simulink model "quad_new_leg_raibert_strategy_v2"  (R2022b)
settings: Solver=ode15s  StartTime=0.0  StopTime=40  RelTol=1e-3
InitFcn:
  | init_quad_new_leg_raibert_strategy_v2
undefined symbols (not defined in the file): body, ctrl, Extr_Data_LinkEndHole, ground, l1, l2, m1, m2, planner, X, Y, Z
libraries: sm_lib x114, nesl_utility x74, slpidlib x24, simulink x5, Contact_Forces_Lib x4, Parts_Lib x4, sharedtransform x2
(part 1 of 7)
settings Model: Creator=biorobotics  LastModifiedBy=sheri
settings SolverCC: AlgebraicLoopSolver=TrustRegion
settings DataIOCC: ReturnWorkspaceOutputs=off
settings DebuggingCC: UnconnectedInputMsg=warning  UnconnectedOutputMsg=warning  UnconnectedLineMsg=warning  SFMachineParentedDataDiag=warning  ArithmeticOperatorsInVariantConditions=warning
settings ModelReferenceCC: EnableRefExpFcnMdlSchedulingChecks=on
settings SFSimCC: SimUseLocalCustomCode=off  CustomCodeUndefinedFunction=UseInterfaceOnly
settings RTWCC: RTWUseLocalCustomCode=off
settings DiagnosticsConfigSet: SimMechanicsRigidlyBoundBlock=none

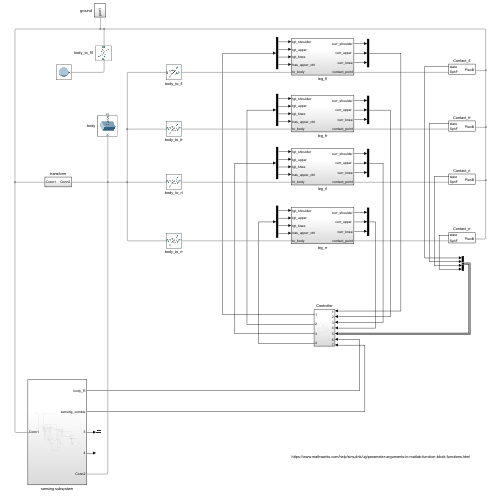
[thumbnail: Simulink's stored preview of the top-level diagram]
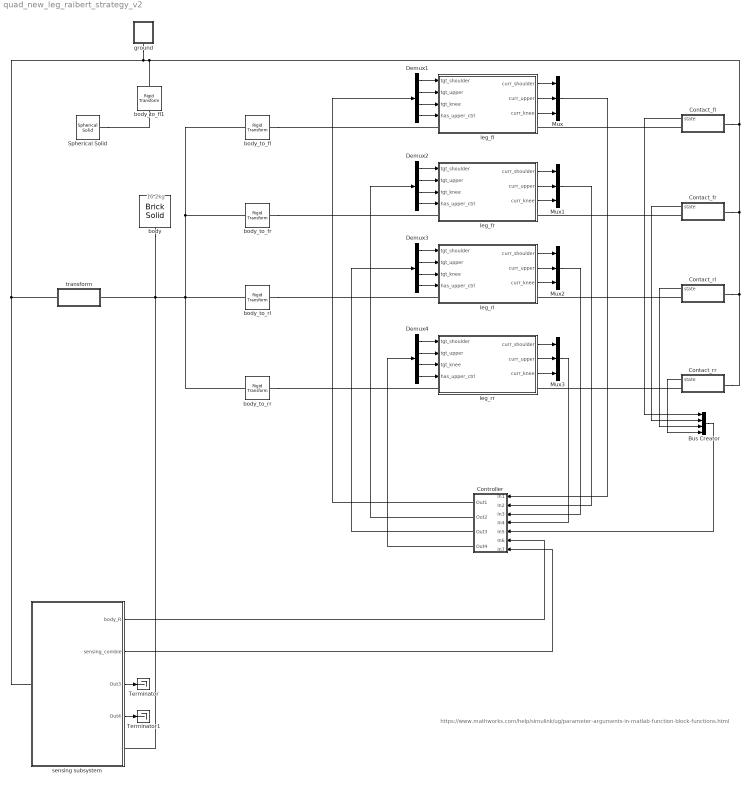
== system quad_new_leg_raibert_strategy_v2 ==
  note: https://www.mathworks.com/help/simulink/ug/parameter-arguments-in-matlab-function-block-functions.html
  note: 16.2kg
  Bus Creator : BusCreator  Inputs=4
  Contact_fl : Subsystem
  Contact_fr : Subsystem
  Contact_rl : Subsystem
  Contact_rr : Subsystem
  Controller : Subsystem
  Demux{1..4} (4 alike) : Demux
  Mux{,1..3} (4 alike) : Mux  Inputs=3
  Spherical Solid : sm_lib/Body Elements/Spherical Solid  GraphicAmbientColor=[0.15 0.15 0.15 1.0]  BasedOnType=Density  CenterOfMass=[0 0 0]  CenterOfMassUnits=m  GraphicDiffuseColor=[0.4 0.2 0.0]  Density=1000  DensityUnits=kg/m^3  DoExposeReferenceFrame=on  GraphicEmissiveColor=[0.0 0.0 0.0 1.0]  ExportEntireGeometry=off  SerializedExposedGeometries=<ExposedGeometries/>  SerializedFrames=<Frames/>  MarkerShape=Sphere  MarkerSize=10  GraphicType=FromGeometry  InertiaType=CalculateFromGeometry  Mass=1  MassUnits=kg  MomentsOfInertia=[1 1 1]  MomentsOfInertiaUnits=kg*m^2  GraphicOpacity=1.0  ProductsOfInertia=[0 0 0]  ProductsOfInertiaUnits=kg*m^2  GraphicShininess=75  GraphicSpecularColor=[0.5 0.5 0.5 1.0]  SphereRadius=0.1  SphereRadiusUnits=m  GraphicVisPropType=SimpleVisualProperties
  Terminator : Terminator
  Terminator1 : Terminator
  body : sm_lib/Body Elements/Brick Solid  GraphicAmbientColor=[0.15 0.15 0.15 1.0]  BasedOnType=Density  BrickDimensions=[body.x_length body.y_length body.z_length]  BrickDimensionUnits=m  CenterOfMass=[0 0 0]  CenterOfMassUnits=m  GraphicDiffuseColor=[164 184 200]/255  Density=600  DensityUnits=kg/(m^3)  DoExposeReferenceFrame=on  GraphicEmissiveColor=[0.0 0.0 0.0 1.0]  ExportEntireGeometry=off  SerializedFrames=<Frames><Frame><Id>Frame2</Id><Value><Name>force</Name><Origin><Source>CenterOfMassFrame</Source><FeatureName></FeatureName></Origin><PrimaryAxis><DefinedDirection>+Z</DefinedDirection><Source>ReferenceFrame</Source><SourceDirection>+Z</SourceDirection><FeatureName></FeatureName></PrimaryAxis><SecondaryAxis><DefinedDirection>+X</DefinedDirection><Source>ReferenceFrame</Source><SourceDirection>+X</SourceDirection><FeatureName></FeatureName></SecondaryAxis></Value></Frame></Frames>  MarkerShape=Sphere  MarkerSize=10  GraphicType=FromGeometry  InertiaType=CalculateFromGeometry  Mass=8.6  MassUnits=kg  MomentsOfInertia=[1 1 1]  MomentsOfInertiaUnits=kg*m^2  GraphicOpacity=1.0  ProductsOfInertia=[0 0 0]  ProductsOfInertiaUnits=kg*m^2  GraphicShininess=75  GraphicSpecularColor=[0.5 0.5 0.5 1.0]  GraphicVisPropType=SimpleVisualProperties
  body_to_fl : sm_lib/Frames and Transforms/Rigid Transform  TranslationMethod=Cartesian  TranslationStandardOffset=0  TranslationLengthUnit=m  TranslationStandardAxis=+Z  TranslationCartesianOffset=[body.shoulder_distance body.y_length/2+body.shoulder_size/2 0]  TranslationROffset=0  TranslationROffsetUnits=m  TranslationZOffset=0  TranslationZOffsetUnits=m  TranslationThetaOffset=0  TranslationThetaOffsetUnits=deg  RotationMethod=AlignedAxes  RotationAngleUnits=deg  RotationStandardAxis=+Z  RotationAngle=0.0  RotationArbitraryAxis=[0 0 1]  FollAlignAxisA=+Z  BaseAlignAxisA=+X  FollAlignAxisB=+X  BaseAlignAxisB=-Z  RotationSequenceAxes=FollowerAxes  RotationSequence=XYX  RotationSequenceAngles=[0 0 0]  RotationSequenceAnglesUnits=deg  RotationMatrix=[1 0 0; 0 1 0; 0 0 1]  Quaternion=[1 0 0 0]
  body_to_fl1 : sm_lib/Frames and Transforms/Rigid Transform  TranslationMethod=Cartesian  TranslationStandardOffset=0  TranslationLengthUnit=m  TranslationStandardAxis=+Z  TranslationCartesianOffset=[5 5 0]  TranslationROffset=0  TranslationROffsetUnits=m  TranslationZOffset=0  TranslationZOffsetUnits=m  TranslationThetaOffset=0  TranslationThetaOffsetUnits=deg  RotationMethod=None  RotationAngleUnits=deg  RotationStandardAxis=+Z  RotationAngle=0.0  RotationArbitraryAxis=[0 0 1]  FollAlignAxisA=+Z  BaseAlignAxisA=+X  FollAlignAxisB=+X  BaseAlignAxisB=-Z  RotationSequenceAxes=FollowerAxes  RotationSequence=XYX  RotationSequenceAngles=[0 0 0]  RotationSequenceAnglesUnits=deg  RotationMatrix=[1 0 0; 0 1 0; 0 0 1]  Quaternion=[1 0 0 0]
  body_to_fr : sm_lib/Frames and Transforms/Rigid Transform  TranslationMethod=Cartesian  TranslationStandardOffset=0  TranslationLengthUnit=m  TranslationStandardAxis=+Z  TranslationCartesianOffset=[body.shoulder_distance -body.y_length/2-body.shoulder_size/2 0]  TranslationROffset=0  TranslationROffsetUnits=m  TranslationZOffset=0  TranslationZOffsetUnits=m  TranslationThetaOffset=0  TranslationThetaOffsetUnits=deg  RotationMethod=AlignedAxes  RotationAngleUnits=deg  RotationStandardAxis=+Z  RotationAngle=0.0  RotationArbitraryAxis=[0 0 1]  FollAlignAxisA=+Z  BaseAlignAxisA=+X  FollAlignAxisB=+X  BaseAlignAxisB=-Z  RotationSequenceAxes=FollowerAxes  RotationSequence=XYX  RotationSequenceAngles=[0 0 0]  RotationSequenceAnglesUnits=deg  RotationMatrix=[1 0 0; 0 1 0; 0 0 1]  Quaternion=[1 0 0 0]
  body_to_rl : sm_lib/Frames and Transforms/Rigid Transform  TranslationMethod=Cartesian  TranslationStandardOffset=0  TranslationLengthUnit=m  TranslationStandardAxis=+Z  TranslationCartesianOffset=[-body.shoulder_distance body.y_length/2+body.shoulder_size/2 0]  TranslationROffset=0  TranslationROffsetUnits=m  TranslationZOffset=0  TranslationZOffsetUnits=m  TranslationThetaOffset=0  TranslationThetaOffsetUnits=deg  RotationMethod=AlignedAxes  RotationAngleUnits=deg  RotationStandardAxis=+Z  RotationAngle=0.0  RotationArbitraryAxis=[0 0 1]  FollAlignAxisA=+Z  BaseAlignAxisA=+X  FollAlignAxisB=+X  BaseAlignAxisB=-Z  RotationSequenceAxes=FollowerAxes  RotationSequence=XYX  RotationSequenceAngles=[0 0 0]  RotationSequenceAnglesUnits=deg  RotationMatrix=[1 0 0; 0 1 0; 0 0 1]  Quaternion=[1 0 0 0]
  body_to_rr : sm_lib/Frames and Transforms/Rigid Transform  TranslationMethod=Cartesian  TranslationStandardOffset=0  TranslationLengthUnit=m  TranslationStandardAxis=+Z  TranslationCartesianOffset=[-body.shoulder_distance -body.y_length/2-body.shoulder_size/2 0]  TranslationROffset=0  TranslationROffsetUnits=m  TranslationZOffset=0  TranslationZOffsetUnits=m  TranslationThetaOffset=0  TranslationThetaOffsetUnits=deg  RotationMethod=AlignedAxes  RotationAngleUnits=deg  RotationStandardAxis=+Z  RotationAngle=0.0  RotationArbitraryAxis=[0 0 1]  FollAlignAxisA=+Z  BaseAlignAxisA=+X  FollAlignAxisB=+X  BaseAlignAxisB=-Z  RotationSequenceAxes=FollowerAxes  RotationSequence=XYX  RotationSequenceAngles=[0 0 0]  RotationSequenceAnglesUnits=deg  RotationMatrix=[1 0 0; 0 1 0; 0 0 1]  Quaternion=[1 0 0 0]
  ground : Subsystem
  leg_fl : Subsystem
  leg_fr : Subsystem
  leg_rl : Subsystem
  leg_rr : Subsystem
  "sensing subsystem " : Subsystem
  transform : Subsystem
  wires:
  leg_fl/1(curr_shoulder) -> Mux/1
  leg_fl/2("curr_upper ") -> Mux/2
  leg_fl/3(curr_knee) -> Mux/3
  leg_fr/2("curr_upper ") -> Mux1/2
  leg_fr/1(curr_shoulder) -> Mux1/1
  leg_fr/3(curr_knee) -> Mux1/3
  leg_rl/1(curr_shoulder) -> Mux2/1
  leg_rl/2("curr_upper ") -> Mux2/2
  leg_rl/3(curr_knee) -> Mux2/3
  leg_rr/1(curr_shoulder) -> Mux3/1
  leg_rr/2("curr_upper ") -> Mux3/2
  leg_rr/3(curr_knee) -> Mux3/3
  Contact_fl/1(state) -> Bus Creator/1
  Contact_rr/1(state) -> Bus Creator/4
  Contact_rl/1(state) -> Bus Creator/3
  Contact_fr/1(state) -> Bus Creator/2
  Demux1/1 -> leg_fl/1(tgt_shoulder)
  Demux1/3 -> leg_fl/3(tgt_knee)
  Demux1/2 -> leg_fl/2(tgt_upper)
  Demux1/4 -> leg_fl/4(has_upper_ctrl)
  Demux2/1 -> leg_fr/1(tgt_shoulder)
  Demux2/3 -> leg_fr/3(tgt_knee)
  Demux2/4 -> leg_fr/4(has_upper_ctrl)
  Demux2/2 -> leg_fr/2(tgt_upper)
  Demux3/4 -> leg_rl/4(has_upper_ctrl)
  Demux3/3 -> leg_rl/3(tgt_knee)
  Demux3/1 -> leg_rl/1(tgt_shoulder)
  Demux3/2 -> leg_rl/2(tgt_upper)
  Demux4/1 -> leg_rr/1(tgt_shoulder)
  Demux4/2 -> leg_rr/2(tgt_upper)
  Demux4/3 -> leg_rr/3(tgt_knee)
  Demux4/4 -> leg_rr/4(has_upper_ctrl)
  Mux/1 -> Controller/1(In1)
  Mux1/1 -> Controller/2(In2)
  Mux2/1 -> Controller/3(In3)
  Mux3/1 -> Controller/4(In4)
  Bus Creator/1 -> Controller/5(In5)
  "sensing subsystem "/1(body_R) -> Controller/6(In6)
  "sensing subsystem "/2(sensing_combie) -> Controller/7(In7)
  Controller/1(Out1) -> Demux1/1
  Controller/2(Out2) -> Demux2/1
  Controller/3(Out3) -> Demux3/1
  Controller/4(Out4) -> Demux4/1
  "sensing subsystem "/3(Out3) -> Terminator/1
  "sensing subsystem "/4(Out4) -> Terminator1/1
  connections:
  body_to_fl/RConn1 -- leg_fl/LConn1
  body_to_rl/RConn1 -- leg_rl/LConn1
  Contact_fl/RConn1 -- leg_fl/RConn1
  Contact_fr/RConn1 -- leg_fr/RConn1
  Contact_rl/RConn1 -- leg_rl/RConn1
  Contact_rr/RConn1 -- leg_rr/RConn1
  body_to_rr/RConn1 -- leg_rr/LConn1
  body_to_fr/RConn1 -- leg_fr/LConn1
  Spherical Solid/RConn1 -- body_to_fl1/RConn1
  Contact_fr/LConn1 -- body_to_fl1/LConn1 -- transform/RConn1 -- "sensing subsystem "/LConn1 -- ground/RConn1 -- Contact_fl/LConn1 -- Contact_rr/LConn1 -- Contact_rl/LConn1
  body_to_rl/LConn1 -- body_to_rr/LConn1 -- body_to_fl/LConn1 -- body_to_fr/LConn1 -- transform/LConn1 -- body/RConn1 -- "sensing subsystem "/RConn1

== system quad_new_leg_raibert_strategy_v2/Contact_fl ==
  note: state 4 166.31ms
  note: 这是一个蛋疼的处理，因为地面现在厚度是0.4，为了和碰撞的block要求匹配，所以碰撞是相对于这个地面的中心来算的。而检测高度的时候就要把这个厚度减掉
      | 但是Transform sensor要检测的是球和地面的高度差
  Bus Selector : BusSelector  OutputSignals=Normal Force,Frame Sep,Friction Force
  Compare To Constant : simulink/Logic and Bit Operations/Compare To Constant  relop=<=  const=planner.touch_down_height  OutDataTypeStr=uint8
  PSConv4 : nesl_utility/PS-Simulink Converter  PhysicalDomain=network_engine_domain  SubClassName=ps_output  LeftPortType=input  RightPortType=output  PseudoPeriodic=off  Frequencies=[]  VectorFormat=1-D array  Unit=1  AffineConversion=off
  Sphere to Plane Force1 : Contact_Forces_Lib/3D/Sphere to Plane Force  sphere_rad=body.foot_radius  plane_lenx=12  plane_leny=12  plane_depth=0  force_law=Linear  k_contact=ground.stiff  b_contact=ground.damp  pen_full_damp_F=1e-4  pen_exponent=1  custom_param_1=1  custom_param_2=1  friction_law=Stick-Slip Continuous  mu_kinetic=0.7  mu_static=0.7  v_thr=0.001
  State Scope : Scope
  Terminator : Terminator
  Transform Sensor : sm_lib/Frames and Transforms/Transform Sensor  MeasurementFrame=World  SenseAngle=off  SenseAxis=off  SenseQ=off  SenseR=off  SenseRotationSequence=off  RotationSequence=XYX  SenseOmegaX=off  SenseOmegaY=off  SenseOmegaZ=off  SenseQDot=off  SenseRDot=off  SenseAlphaX=off  SenseAlphaY=off  SenseAlphaZ=off  SenseQDDot=off  SenseRDDot=off  SenseX=off  SenseY=off  SenseZ=on  SenseRad=off  SenseAzim=off  SenseDist=off  SenseInc=off  SenseXDot=off  SenseYDot=off  SenseZDot=off  SenseRadDot=off  SenseAzimDot=off  SenseDistDot=off  SenseIncDot=off  SenseXDDot=off  SenseYDDot=off  SenseZDDot=off  SenseRadDDot=off  SenseAzimDDot=off  SenseDistDDot=off  SenseIncDDot=off
  ZScope : Scope
  force : Scope  NumInputPorts=2
  PlanB : PMIOPort  Side=Left
  SphF : PMIOPort  Port=2  Side=Right
  state : Outport  VectorParamsAs1DForOutWhenUnconnected=off
  wires:
  Sphere to Plane Force1/1 -> Bus Selector/1
  Bus Selector/1 -> force/1  "<Normal Force>"
  PSConv4/1 -> Compare To Constant/1, ZScope/1
  Compare To Constant/1 -> state/1, State Scope/1
  Bus Selector/3 -> force/2  "<Friction Force>"
  Bus Selector/2 -> Terminator/1  "<Frame Sep>"
  connections:
  Sphere to Plane Force1/LConn1 -- Transform Sensor/RConn1 -- SphF/RConn1
  Sphere to Plane Force1/RConn1 -- Transform Sensor/LConn1 -- PlanB/RConn1
  PSConv4/LConn1 -- Transform Sensor/RConn2

== system quad_new_leg_raibert_strategy_v2/Contact_fr ==
  note: state 4 166.31ms
  note: 这是一个蛋疼的处理，因为地面现在厚度是0.4，为了和碰撞的block要求匹配，所以碰撞是相对于这个地面的中心来算的。而检测高度的时候就要把这个厚度减掉
      | 但是Transform sensor要检测的是球和地面的高度差
  Bus Selector : BusSelector  OutputSignals=Normal Force,Frame Sep,Friction Force
  Compare To Constant : simulink/Logic and Bit Operations/Compare To Constant  relop=<=  const=planner.touch_down_height  OutDataTypeStr=uint8
  PSConv4 : nesl_utility/PS-Simulink Converter  PhysicalDomain=network_engine_domain  SubClassName=ps_output  LeftPortType=input  RightPortType=output  PseudoPeriodic=off  Frequencies=[]  VectorFormat=1-D array  Unit=1  AffineConversion=off
  Sphere to Plane Force1 : Contact_Forces_Lib/3D/Sphere to Plane Force  sphere_rad=body.foot_radius  plane_lenx=12  plane_leny=12  plane_depth=0  force_law=Linear  k_contact=ground.stiff  b_contact=ground.damp  pen_full_damp_F=1e-4  pen_exponent=1  custom_param_1=1  custom_param_2=1  friction_law=Stick-Slip Continuous  mu_kinetic=0.7  mu_static=0.7  v_thr=0.001
  State Scope : Scope
  Terminator : Terminator
  Transform Sensor : sm_lib/Frames and Transforms/Transform Sensor  MeasurementFrame=World  SenseAngle=off  SenseAxis=off  SenseQ=off  SenseR=off  SenseRotationSequence=off  RotationSequence=XYX  SenseOmegaX=off  SenseOmegaY=off  SenseOmegaZ=off  SenseQDot=off  SenseRDot=off  SenseAlphaX=off  SenseAlphaY=off  SenseAlphaZ=off  SenseQDDot=off  SenseRDDot=off  SenseX=off  SenseY=off  SenseZ=on  SenseRad=off  SenseAzim=off  SenseDist=off  SenseInc=off  SenseXDot=off  SenseYDot=off  SenseZDot=off  SenseRadDot=off  SenseAzimDot=off  SenseDistDot=off  SenseIncDot=off  SenseXDDot=off  SenseYDDot=off  SenseZDDot=off  SenseRadDDot=off  SenseAzimDDot=off  SenseDistDDot=off  SenseIncDDot=off
  ZScope : Scope
  force : Scope  NumInputPorts=2
  PlanB : PMIOPort  Side=Left
  SphF : PMIOPort  Port=2  Side=Right
  state : Outport  VectorParamsAs1DForOutWhenUnconnected=off
  wires:
  Sphere to Plane Force1/1 -> Bus Selector/1
  Bus Selector/1 -> force/1  "<Normal Force>"
  PSConv4/1 -> Compare To Constant/1, ZScope/1
  Compare To Constant/1 -> state/1, State Scope/1
  Bus Selector/3 -> force/2  "<Friction Force>"
  Bus Selector/2 -> Terminator/1  "<Frame Sep>"
  connections:
  Sphere to Plane Force1/LConn1 -- Transform Sensor/RConn1 -- SphF/RConn1
  Sphere to Plane Force1/RConn1 -- Transform Sensor/LConn1 -- PlanB/RConn1
  PSConv4/LConn1 -- Transform Sensor/RConn2

== system quad_new_leg_raibert_strategy_v2/Contact_rl ==
  note: 这是一个蛋疼的处理，因为地面现在厚度是0.4，为了和碰撞的block要求匹配，所以碰撞是相对于这个地面的中心来算的。而检测高度的时候就要把这个厚度减掉
      | 但是Transform sensor要检测的是球和地面的高度差
  Bus Selector : BusSelector  OutputSignals=Normal Force,Frame Sep,Friction Force
  Compare To Constant : simulink/Logic and Bit Operations/Compare To Constant  relop=<=  const=planner.touch_down_height  OutDataTypeStr=uint8
  PSConv4 : nesl_utility/PS-Simulink Converter  PhysicalDomain=network_engine_domain  SubClassName=ps_output  LeftPortType=input  RightPortType=output  PseudoPeriodic=off  Frequencies=[]  VectorFormat=1-D array  Unit=1  AffineConversion=off
  Sphere to Plane Force1 : Contact_Forces_Lib/3D/Sphere to Plane Force  sphere_rad=body.foot_radius  plane_lenx=12  plane_leny=12  plane_depth=0  force_law=Linear  k_contact=ground.stiff  b_contact=ground.damp  pen_full_damp_F=1e-4  pen_exponent=1  custom_param_1=1  custom_param_2=1  friction_law=Stick-Slip Continuous  mu_kinetic=0.7  mu_static=0.7  v_thr=0.001
  State Scope : Scope
  Terminator : Terminator
  Transform Sensor : sm_lib/Frames and Transforms/Transform Sensor  MeasurementFrame=World  SenseAngle=off  SenseAxis=off  SenseQ=off  SenseR=off  SenseRotationSequence=off  RotationSequence=XYX  SenseOmegaX=off  SenseOmegaY=off  SenseOmegaZ=off  SenseQDot=off  SenseRDot=off  SenseAlphaX=off  SenseAlphaY=off  SenseAlphaZ=off  SenseQDDot=off  SenseRDDot=off  SenseX=off  SenseY=off  SenseZ=on  SenseRad=off  SenseAzim=off  SenseDist=off  SenseInc=off  SenseXDot=off  SenseYDot=off  SenseZDot=off  SenseRadDot=off  SenseAzimDot=off  SenseDistDot=off  SenseIncDot=off  SenseXDDot=off  SenseYDDot=off  SenseZDDot=off  SenseRadDDot=off  SenseAzimDDot=off  SenseDistDDot=off  SenseIncDDot=off
  ZScope : Scope
  force : Scope  NumInputPorts=2
  PlanB : PMIOPort  Side=Left
  SphF : PMIOPort  Port=2  Side=Right
  state : Outport  VectorParamsAs1DForOutWhenUnconnected=off
  wires:
  Sphere to Plane Force1/1 -> Bus Selector/1
  Bus Selector/1 -> force/1  "<Normal Force>"
  PSConv4/1 -> Compare To Constant/1, ZScope/1
  Compare To Constant/1 -> state/1, State Scope/1
  Bus Selector/3 -> force/2  "<Friction Force>"
  Bus Selector/2 -> Terminator/1  "<Frame Sep>"
  connections:
  Sphere to Plane Force1/LConn1 -- Transform Sensor/RConn1 -- SphF/RConn1
  Sphere to Plane Force1/RConn1 -- Transform Sensor/LConn1 -- PlanB/RConn1
  PSConv4/LConn1 -- Transform Sensor/RConn2

== system quad_new_leg_raibert_strategy_v2/Contact_rr ==
  note: state 4 166.31ms
  note: 这是一个蛋疼的处理，因为地面现在厚度是0.4，为了和碰撞的block要求匹配，所以碰撞是相对于这个地面的中心来算的。而检测高度的时候就要把这个厚度减掉
      | 但是Transform sensor要检测的是球和地面的高度差
  Bus Selector : BusSelector  OutputSignals=Normal Force,Frame Sep,Friction Force
  Compare To Constant : simulink/Logic and Bit Operations/Compare To Constant  relop=<=  const=planner.touch_down_height  OutDataTypeStr=uint8
  PSConv4 : nesl_utility/PS-Simulink Converter  PhysicalDomain=network_engine_domain  SubClassName=ps_output  LeftPortType=input  RightPortType=output  PseudoPeriodic=off  Frequencies=[]  VectorFormat=1-D array  Unit=1  AffineConversion=off
  Sphere to Plane Force1 : Contact_Forces_Lib/3D/Sphere to Plane Force  sphere_rad=body.foot_radius  plane_lenx=12  plane_leny=12  plane_depth=0  force_law=Linear  k_contact=ground.stiff  b_contact=ground.damp  pen_full_damp_F=1e-4  pen_exponent=1  custom_param_1=1  custom_param_2=1  friction_law=Stick-Slip Continuous  mu_kinetic=0.7  mu_static=0.7  v_thr=0.001
  State Scope : Scope
  Terminator : Terminator
  Transform Sensor : sm_lib/Frames and Transforms/Transform Sensor  MeasurementFrame=World  SenseAngle=off  SenseAxis=off  SenseQ=off  SenseR=off  SenseRotationSequence=off  RotationSequence=XYX  SenseOmegaX=off  SenseOmegaY=off  SenseOmegaZ=off  SenseQDot=off  SenseRDot=off  SenseAlphaX=off  SenseAlphaY=off  SenseAlphaZ=off  SenseQDDot=off  SenseRDDot=off  SenseX=off  SenseY=off  SenseZ=on  SenseRad=off  SenseAzim=off  SenseDist=off  SenseInc=off  SenseXDot=off  SenseYDot=off  SenseZDot=off  SenseRadDot=off  SenseAzimDot=off  SenseDistDot=off  SenseIncDot=off  SenseXDDot=off  SenseYDDot=off  SenseZDDot=off  SenseRadDDot=off  SenseAzimDDot=off  SenseDistDDot=off  SenseIncDDot=off
  ZScope : Scope
  force : Scope  NumInputPorts=2
  PlanB : PMIOPort  Side=Left
  SphF : PMIOPort  Port=2  Side=Right
  state : Outport  VectorParamsAs1DForOutWhenUnconnected=off
  wires:
  Sphere to Plane Force1/1 -> Bus Selector/1
  Bus Selector/1 -> force/1  "<Normal Force>"
  PSConv4/1 -> Compare To Constant/1, ZScope/1
  Compare To Constant/1 -> state/1, State Scope/1
  Bus Selector/3 -> force/2  "<Friction Force>"
  Bus Selector/2 -> Terminator/1  "<Frame Sep>"
  connections:
  Sphere to Plane Force1/LConn1 -- Transform Sensor/RConn1 -- SphF/RConn1
  Sphere to Plane Force1/RConn1 -- Transform Sensor/LConn1 -- PlanB/RConn1
  PSConv4/LConn1 -- Transform Sensor/RConn2

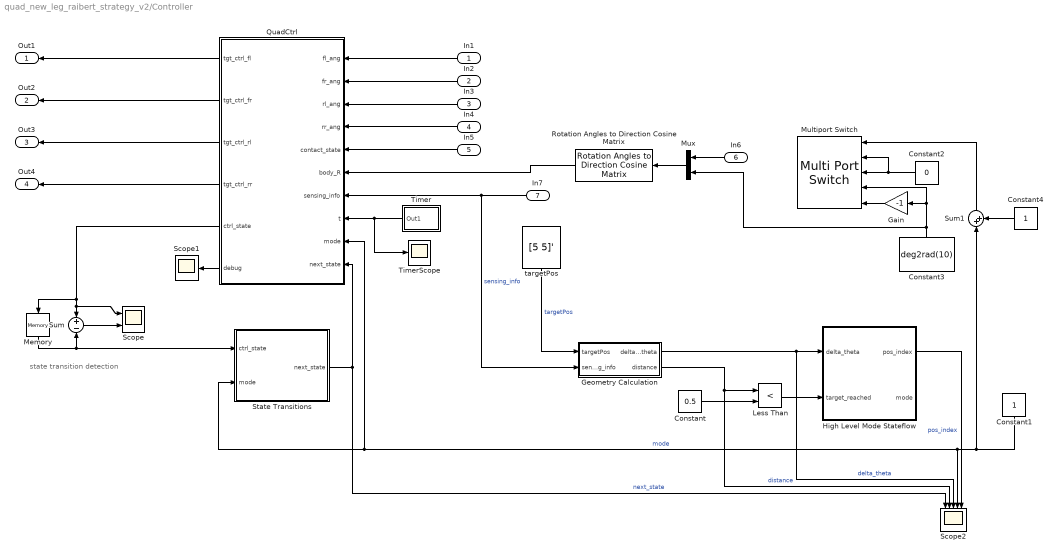
== system quad_new_leg_raibert_strategy_v2/Controller ==
  note: state transition detection
  In1 : Inport
  In2 : Inport  Port=2
  In3 : Inport  Port=3
  In4 : Inport  Port=4
  In5 : Inport  Port=5
  In6 : Inport  Port=6
  In7 : Inport  Port=7
  Constant : Constant  Value=0.5
  Constant1 : Constant
  Constant2 : Constant  Value=0
  Constant3 : Constant  Value=deg2rad(10)
  Constant4 : Constant
  Gain : Gain  Gain=-1
  Geometry Calculation : Subsystem
  High Level Mode Stateflow : Stateflow chart  TreatAsAtomicUnit=on
      settings: PortSchema="{\"entries\":[{\"content\":{\"sides\":[{\"content\":{\"connectorIds\":[\"In2\",\"In1\"]},\"type\":\"ConnectorPlacement.EquallySpacedRectSide\",\"uuid\":\"54635eaa-af22-4c07-946c-8b3764ca4079\"},{\"content\":{\"connectorIds\":[\"Out1\",\"Out2\"],\"side\":\"RIGHT\"},\"type\":\"ConnectorPlacement.EquallySpacedRectSide\",\"uuid\":\"b8ca9e50-c21e-481d-aebe-d3447dd5b6ec\"},{\"content\":{\"connectorIds\":[],\"side\":\"TOP\"},\"type\":\"ConnectorPlacement.EquallySpacedRectSide\",\"uuid\":\"aa364018-0c1f-4137-8fa7-722b902e07a1\"}]},\"type\":\"ConnectorPlacement.EquallySpacedConnector\",\"uuid\":\"b87c06e7-bef4-4368-b066-66035be64295\"}],\"packageUris\":[\"http://schema.mathworks.com/mf0/Connector/R2020b\"],\"version\":\"1.0\"}"
  Less Than : RelationalOperator  Operator=<  OutDataTypeStr=boolean  RndMeth=Simplest  InputSameDT=off
  Memory : Memory
  Multiport Switch : MultiPortSwitch  Inputs=4  SaturateOnIntegerOverflow=off  InputSameDT=off
  Mux : Mux  Inputs=2
  QuadCtrl : MATLAB Function  TreatAsAtomicUnit=on  SystemSampleTime=0.0025
  Rotation Angles to Direction Cosine Matrix : sharedtransform/Rotation Angles to Direction Cosine Matrix  rotationOrder=XYZ  aMode=aMode
  Scope : Scope  NumInputPorts=2
  Scope1 : Scope
  Scope2 : Scope  NumInputPorts=5
  State Transitions : Stateflow chart  TreatAsAtomicUnit=on
  Sum : Sum  Inputs=+-
  Sum1 : Sum  Inputs=|++
  Timer : Subsystem
  TimerScope : Scope
  targetPos : Constant  Value=[5 5]'  VectorParams1D=off
  Out1 : Outport  VectorParamsAs1DForOutWhenUnconnected=off
  Out2 : Outport  Port=2  VectorParamsAs1DForOutWhenUnconnected=off
  Out3 : Outport  Port=3  VectorParamsAs1DForOutWhenUnconnected=off
  Out4 : Outport  Port=4  VectorParamsAs1DForOutWhenUnconnected=off
  wires:
  In7/1 -> Geometry Calculation/2(sensing_info), QuadCtrl/7(sensing_info)  "sensing_info"
  In4/1 -> QuadCtrl/4(rr_ang)
  Timer/1(Out1) -> TimerScope/1, QuadCtrl/8(t)
  In3/1 -> QuadCtrl/3(rl_ang)
  In5/1 -> QuadCtrl/5(contact_state)
  In1/1 -> QuadCtrl/1(fl_ang)
  QuadCtrl/3(tgt_ctrl_rl) -> Out3/1
  In6/1 -> Mux/1
  QuadCtrl/2(tgt_ctrl_fr) -> Out2/1
  In2/1 -> QuadCtrl/2(fr_ang)
  QuadCtrl/4(tgt_ctrl_rr) -> Out4/1
  QuadCtrl/1(tgt_ctrl_fl) -> Out1/1
  QuadCtrl/5(ctrl_state) -> Scope/1, Sum/1, Memory/1
  Memory/1 -> State Transitions/1(ctrl_state), Sum/2
  Sum/1 -> Scope/2
  QuadCtrl/6(debug) -> Scope1/1
  Less Than/1 -> High Level Mode Stateflow/1(target_reached)
  Constant1/1 -> Sum1/1, State Transitions/2(mode), QuadCtrl/9(mode), Scope2/4  "mode"
  Constant/1 -> Less Than/2
  State Transitions/1(next_state) -> Scope2/1, QuadCtrl/10(next_state)  "next_state"
  Geometry Calculation/2(distance) -> Scope2/2, Less Than/1  "distance"
  Geometry Calculation/1(delta_theta) -> Scope2/3, High Level Mode Stateflow/2(delta_theta)  "delta_theta"
  targetPos/1 -> Geometry Calculation/1(targetPos)  "targetPos"
  High Level Mode Stateflow/1(pos_index) -> Scope2/5  "pos_index"
  Mux/1 -> Rotation Angles to Direction Cosine Matrix/1
  Rotation Angles to Direction Cosine Matrix/1 -> QuadCtrl/6(body_R)
  Constant2/1 -> Multiport Switch/2, Multiport Switch/3
  Constant3/1 -> Mux/2, Gain/1, Multiport Switch/4
  Sum1/1 -> Multiport Switch/1
  Constant4/1 -> Sum1/2
  Gain/1 -> Multiport Switch/5

== system quad_new_leg_raibert_strategy_v2/ground ==
  Mechanism Configuration : sm_lib/Utilities/Mechanism Configuration  UniformGravity=Constant  GravityVector=[0 0 -9.80665]  GravityUnits=m/s^2  LinearizationDelta=0.001  JointModeTransitionNonlinearIterations=2
  Rigid Transform : sm_lib/Frames and Transforms/Rigid Transform  TranslationMethod=StandardAxis  TranslationStandardOffset=ground.height/2  TranslationLengthUnit=m  TranslationStandardAxis=+Z  TranslationCartesianOffset=[0 0 0]  TranslationROffset=0  TranslationROffsetUnits=m  TranslationZOffset=0  TranslationZOffsetUnits=m  TranslationThetaOffset=0  TranslationThetaOffsetUnits=deg  RotationMethod=None  RotationAngleUnits=deg  RotationStandardAxis=+Z  RotationAngle=0.0  RotationArbitraryAxis=[0 0 1]  FollAlignAxisA=+X  BaseAlignAxisA=+Y  FollAlignAxisB=+Y  BaseAlignAxisB=+Z  RotationSequenceAxes=FollowerAxes  RotationSequence=XYX  RotationSequenceAngles=[0 0 0]  RotationSequenceAnglesUnits=deg  RotationMatrix=[1 0 0; 0 1 0; 0 0 1]  Quaternion=[1 0 0 0]
  Solver Configuration : nesl_utility/Solver Configuration  PhysicalDomain=network_engine_domain  SubClassName=solver  LeftPortType=input  RightPortType=generic  Tones=[]  Harmonics=[]  SimulateNoise=off  Profile=off  UseLocalSampling=off  EnableSwitchedLinearOptims=on  FrequencyDomain=off  UseCCode=off  RelTol=0.001  AbsTol=1e-06  MinStep=1e-09  ToWorkspace=off  RevertToSquareIcSolve=off  NumHomotopyIterations=100  PhasorMode=off  PhasorModeNumHarmonics=1  ConsistencySolver=NEWTON_FTOL  IndexReductionMethod=DerivativeReplacement  DoDC=off  ResidualTolerance=1e-09  ConsistencyTolSource=GLOBAL  ConsistencyAbsTol=0.001  ConsistencyRelTol=0.001  ConsistencyTolFactor=0.001  UseLocalSolver=off  LocalSolverChoice=NE_BACKWARD_EULER_ADVANCER  ResolveIndetEquations=on  FunctionEvalNumThread=1  LocalSolverSampleTime=0.001  DoFixedCost=off  MaxNonlinIter=3  MaxModeIter=2  ComputeImpulses=off  ImpulseIterations=2  LinearAlgebra=Sparse  LinearAlgebraNumThread=0  EquationFormulation=NE_TIME_EF  DelaysMemoryBudget=1024  AutomaticFiltering=on  FilteringTimeConstant=0.001  PartitionStorageMethod=AS_NEEDED  PartitionMemoryBudget=1024  PartitionMethod=FAST
  World Frame : sm_lib/Frames and Transforms/World Frame
  ground : sm_lib/Body Elements/Brick Solid  GraphicAmbientColor=[0.15 0.15 0.15 1.0]  BasedOnType=Density  BrickDimensions=[12 12 ground.height]  BrickDimensionUnits=m  CenterOfMass=[0 0 0]  CenterOfMassUnits=m  GraphicDiffuseColor=[0.6 1.0 0.8]  Density=1000  DensityUnits=kg/(m^3)  DoExposeReferenceFrame=on  GraphicEmissiveColor=[0.0 0.0 0.0 1.0]  ExportEntireGeometry=off  SerializedFrames=<Frames/>  MarkerShape=Sphere  MarkerSize=10  GraphicType=FromGeometry  InertiaType=CalculateFromGeometry  Mass=1  MassUnits=kg  MomentsOfInertia=[1 1 1]  MomentsOfInertiaUnits=kg*m^2  GraphicOpacity=1.0  ProductsOfInertia=[0 0 0]  ProductsOfInertiaUnits=kg*m^2  GraphicShininess=75  GraphicSpecularColor=[0.5 0.5 0.5 1.0]  GraphicVisPropType=SimpleVisualProperties
  port1 : PMIOPort  Side=Right
  connections:
  Solver Configuration/RConn1 -- ground/RConn1 -- Mechanism Configuration/RConn1 -- Rigid Transform/LConn1 -- World Frame/RConn1
  port1/RConn1 -- Rigid Transform/RConn1

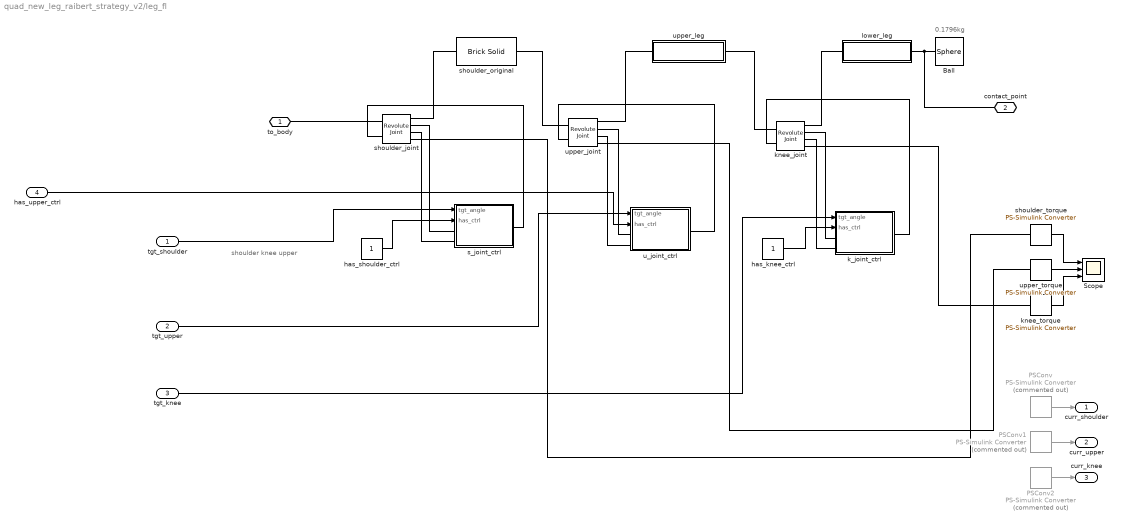
== system quad_new_leg_raibert_strategy_v2/leg_fl ==
  note: 0.1796kg
  note: shoulder knee
      | upper
  tgt_shoulder : Inport
  tgt_upper : Inport  Port=2
  tgt_knee : Inport  Port=3
  has_upper_ctrl : Inport  Port=4
  Ball : Parts_Lib/Sphere  Tag=CustomStyle  sph_radius=body.foot_radius  sph_density=1000  sph_color=red  sph_opacity=1  mark_type=Rings on center planes  arc_width=[40 50]  arc_angle=60  ring_width=5  ring_irad=0.95  mark_color=axes  mark_opacity=1  ring_opacity=0  arc_opacity=0
  PSConv : nesl_utility/PS-Simulink Converter  Commented=on  PhysicalDomain=network_engine_domain  SubClassName=ps_output  LeftPortType=input  RightPortType=output  PseudoPeriodic=off  Frequencies=[]  VectorFormat=1-D array  Unit=1  AffineConversion=off
  PSConv1 : nesl_utility/PS-Simulink Converter  Commented=on  PhysicalDomain=network_engine_domain  SubClassName=ps_output  LeftPortType=input  RightPortType=output  PseudoPeriodic=off  Frequencies=[]  VectorFormat=1-D array  Unit=1  AffineConversion=off
  PSConv2 : nesl_utility/PS-Simulink Converter  Commented=on  PhysicalDomain=network_engine_domain  SubClassName=ps_output  LeftPortType=input  RightPortType=output  PseudoPeriodic=off  Frequencies=[]  VectorFormat=1-D array  Unit=1  AffineConversion=off
  Scope : Scope  NumInputPorts=3
  "has_knee_ctrl " : Constant
  has_shoulder_ctrl : Constant
  k_joint_ctrl : Subsystem
  knee_joint : sm_lib/Joints/Revolute Joint  JointMode=Normal  SenseConstraintForce=off  SenseConstraintForceX=off  SenseConstraintForceY=off  SenseConstraintForceZ=off  SenseConstraintTorque=off  SenseConstraintTorqueX=off  SenseConstraintTorqueY=off  SenseConstraintTorqueZ=off  SenseTotalForce=off  SenseTotalForceX=off  SenseTotalForceY=off  SenseTotalForceZ=off  SenseTotalTorque=off  SenseTotalTorqueX=off  SenseTotalTorqueY=off  SenseTotalTorqueZ=off  CompositeWrenchDir=FollowerOnBase  CompositeWrenchFrame=BaseFrame  EquilibriumPosition=0  EquilibriumPositionUnits=deg  SpringStiffness=0  SpringStiffnessUnits=N*m/rad  DampingCoefficient=body.knee_damping  DampingCoefficientUnits=N*m/(deg/s)  TorqueActuationMode=InputTorque  MotionActuationMode=ComputedMotion  SensePosition=on  SenseVelocity=on  SenseAcceleration=off  SenseTorqueForce=on  SenseLowerLimitTorqueForce=off  SenseUpperLimitTorqueForce=off  LowerLimitSpecify=off  LowerLimitBound=-90  LowerLimitBoundUnits=deg  LowerLimitStiffness=1e4  LowerLimitStiffnessUnits=N*m/deg  LowerLimitDamping=10  LowerLimitDampingUnits=N*m/(deg/s)  LowerLimitTransitionRegionWidth=0.1  LowerLimitTransitionRegionWidthUnits=deg  UpperLimitSpecify=off  UpperLimitBound=90  UpperLimitBoundUnits=deg  UpperLimitStiffness=1e4  UpperLimitStiffnessUnits=N*m/deg  UpperLimitDamping=10  UpperLimitDampingUnits=N*m/(deg/s)  UpperLimitTransitionRegionWidth=0.1  UpperLimitTransitionRegionWidthUnits=deg  PositionTargetSpecify=off  PositionTargetPriority=High  PositionTargetValue=0  PositionTargetValueUnits=deg  VelocityTargetSpecify=off  VelocityTargetPriority=High  VelocityTargetValue=0  VelocityTargetValueUnits=deg/s
  knee_torque : nesl_utility/PS-Simulink Converter  PhysicalDomain=network_engine_domain  SubClassName=ps_output  LeftPortType=input  RightPortType=output  PseudoPeriodic=off  Frequencies=[]  VectorFormat=1-D array  Unit=1  AffineConversion=off
  lower_leg : Subsystem
  "s_joint_ctrl " : Subsystem
  shoulder_joint : sm_lib/Joints/Revolute Joint  JointMode=Normal  SenseConstraintForce=off  SenseConstraintForceX=off  SenseConstraintForceY=off  SenseConstraintForceZ=off  SenseConstraintTorque=off  SenseConstraintTorqueX=off  SenseConstraintTorqueY=off  SenseConstraintTorqueZ=off  SenseTotalForce=off  SenseTotalForceX=off  SenseTotalForceY=off  SenseTotalForceZ=off  SenseTotalTorque=off  SenseTotalTorqueX=off  SenseTotalTorqueY=off  SenseTotalTorqueZ=off  CompositeWrenchDir=FollowerOnBase  CompositeWrenchFrame=BaseFrame  EquilibriumPosition=0  EquilibriumPositionUnits=deg  SpringStiffness=0  SpringStiffnessUnits=N*m/deg  DampingCoefficient=0  DampingCoefficientUnits=N*m/(deg/s)  TorqueActuationMode=InputTorque  MotionActuationMode=ComputedMotion  SensePosition=on  SenseVelocity=on  SenseAcceleration=off  SenseTorqueForce=on  SenseLowerLimitTorqueForce=off  SenseUpperLimitTorqueForce=off  LowerLimitSpecify=off  LowerLimitBound=-90  LowerLimitBoundUnits=deg  LowerLimitStiffness=1e4  LowerLimitStiffnessUnits=N*m/deg  LowerLimitDamping=10  LowerLimitDampingUnits=N*m/(deg/s)  LowerLimitTransitionRegionWidth=0.1  LowerLimitTransitionRegionWidthUnits=deg  UpperLimitSpecify=off  UpperLimitBound=90  UpperLimitBoundUnits=deg  UpperLimitStiffness=1e4  UpperLimitStiffnessUnits=N*m/deg  UpperLimitDamping=10  UpperLimitDampingUnits=N*m/(deg/s)  UpperLimitTransitionRegionWidth=0.1  UpperLimitTransitionRegionWidthUnits=deg  PositionTargetSpecify=off  PositionTargetPriority=High  PositionTargetValue=0  PositionTargetValueUnits=deg  VelocityTargetSpecify=off  VelocityTargetPriority=High  VelocityTargetValue=0  VelocityTargetValueUnits=deg/s
  shoulder_original : sm_lib/Body Elements/Brick Solid  GraphicAmbientColor=[0.15 0.15 0.15 1.0]  BasedOnType=Density  BrickDimensions=[body.shoulder_size body.shoulder_size body.shoulder_size]  BrickDimensionUnits=m  CenterOfMass=[0 0 0]  CenterOfMassUnits=m  GraphicDiffuseColor=[0.2 0.4 0.6]  Density=660  DensityUnits=kg/(m^3)  DoExposeReferenceFrame=off  GraphicEmissiveColor=[0.0 0.0 0.0 1.0]  ExportEntireGeometry=off  SerializedFrames=<Frames><Frame><Id>Frame1</Id><Value><Name>to_body</Name><Origin><Source>CenterOfMassFrame</Source><FeatureName></FeatureName></Origin><PrimaryAxis><DefinedDirection>+Z</DefinedDirection><Source>ReferenceFrame</Source><SourceDirection>+X</SourceDirection><FeatureName></FeatureName></PrimaryAxis><SecondaryAxis><DefinedDirection>+X</DefinedDirection><Source>ReferenceFrame</Source><SourceDirection>-Z</SourceDirection><FeatureName></FeatureName></SecondaryAxis></Value></Frame><Frame><Id>Frame2</Id><Value><Name>to_leg</Name><Origin><Source>ReferenceFrame</Source><FeatureName></FeatureName></Origin><PrimaryAxis><DefinedDirection>+Z</DefinedDirection><Source>ReferenceFrame</Source><SourceDirection>+Y</SourceDirection><FeatureName></FeatureName></PrimaryAxis><SecondaryAxis><DefinedDirection>+X</DefinedDirection><Source>ReferenceFrame</Source><SourceDirection>+X</SourceDirection><FeatureName></FeatureName></SecondaryAxis></Value></Frame></Frames>  MarkerShape=Sphere  MarkerSize=10  GraphicType=FromGeometry  InertiaType=CalculateFromGeometry  Mass=1  MassUnits=kg  MomentsOfInertia=[1 1 1]  MomentsOfInertiaUnits=kg*m^2  GraphicOpacity=1.0  ProductsOfInertia=[0 0 0]  ProductsOfInertiaUnits=kg*m^2  GraphicShininess=75  GraphicSpecularColor=[0.5 0.5 0.5 1.0]  GraphicVisPropType=SimpleVisualProperties
  shoulder_torque : nesl_utility/PS-Simulink Converter  PhysicalDomain=network_engine_domain  SubClassName=ps_output  LeftPortType=input  RightPortType=output  PseudoPeriodic=off  Frequencies=[]  VectorFormat=1-D array  Unit=1  AffineConversion=off
  "u_joint_ctrl " : Subsystem
  upper_joint : sm_lib/Joints/Revolute Joint  JointMode=Normal  SenseConstraintForce=off  SenseConstraintForceX=off  SenseConstraintForceY=off  SenseConstraintForceZ=off  SenseConstraintTorque=off  SenseConstraintTorqueX=off  SenseConstraintTorqueY=off  SenseConstraintTorqueZ=off  SenseTotalForce=off  SenseTotalForceX=off  SenseTotalForceY=off  SenseTotalForceZ=off  SenseTotalTorque=off  SenseTotalTorqueX=off  SenseTotalTorqueY=off  SenseTotalTorqueZ=off  CompositeWrenchDir=FollowerOnBase  CompositeWrenchFrame=BaseFrame  EquilibriumPosition=0  EquilibriumPositionUnits=deg  SpringStiffness=0  SpringStiffnessUnits=N*m/deg  DampingCoefficient=0  DampingCoefficientUnits=N*m/(deg/s)  TorqueActuationMode=InputTorque  MotionActuationMode=ComputedMotion  SensePosition=on  SenseVelocity=on  SenseAcceleration=off  SenseTorqueForce=on  SenseLowerLimitTorqueForce=off  SenseUpperLimitTorqueForce=off  LowerLimitSpecify=off  LowerLimitBound=-90  LowerLimitBoundUnits=deg  LowerLimitStiffness=1e4  LowerLimitStiffnessUnits=N*m/deg  LowerLimitDamping=10  LowerLimitDampingUnits=N*m/(deg/s)  LowerLimitTransitionRegionWidth=0.1  LowerLimitTransitionRegionWidthUnits=deg  UpperLimitSpecify=off  UpperLimitBound=90  UpperLimitBoundUnits=deg  UpperLimitStiffness=1e4  UpperLimitStiffnessUnits=N*m/deg  UpperLimitDamping=10  UpperLimitDampingUnits=N*m/(deg/s)  UpperLimitTransitionRegionWidth=0.1  UpperLimitTransitionRegionWidthUnits=deg  PositionTargetSpecify=off  PositionTargetPriority=High  PositionTargetValue=0  PositionTargetValueUnits=deg  VelocityTargetSpecify=off  VelocityTargetPriority=High  VelocityTargetValue=0  VelocityTargetValueUnits=deg/s
  upper_leg : Subsystem
  upper_torque : nesl_utility/PS-Simulink Converter  PhysicalDomain=network_engine_domain  SubClassName=ps_output  LeftPortType=input  RightPortType=output  PseudoPeriodic=off  Frequencies=[]  VectorFormat=1-D array  Unit=1  AffineConversion=off
  to_body : PMIOPort  Side=Left
  contact_point : PMIOPort  Port=2  Side=Right
  curr_shoulder : Outport  VectorParamsAs1DForOutWhenUnconnected=off
  "curr_upper " : Outport  Port=2  VectorParamsAs1DForOutWhenUnconnected=off
  curr_knee : Outport  Port=3  VectorParamsAs1DForOutWhenUnconnected=off
  wires:
  PSConv/1 -> curr_shoulder/1
  PSConv1/1 -> "curr_upper "/1
  PSConv2/1 -> curr_knee/1
  shoulder_torque/1 -> Scope/1
  upper_torque/1 -> Scope/2
  knee_torque/1 -> Scope/3
  tgt_shoulder/1 -> "s_joint_ctrl "/1(tgt_angle)
  tgt_upper/1 -> "u_joint_ctrl "/1(tgt_angle)
  tgt_knee/1 -> k_joint_ctrl/1(tgt_angle)
  has_shoulder_ctrl/1 -> "s_joint_ctrl "/2(has_ctrl)
  has_upper_ctrl/1 -> "u_joint_ctrl "/2(has_ctrl)
  "has_knee_ctrl "/1 -> k_joint_ctrl/2(has_ctrl)
  connections:
  contact_point/RConn1 -- lower_leg/LConn1 -- Ball/LConn1
  upper_leg/RConn1 -- upper_joint/RConn1
  upper_leg/LConn1 -- knee_joint/LConn1
  lower_leg/RConn1 -- knee_joint/RConn1
  to_body/RConn1 -- shoulder_joint/LConn1
  shoulder_original/RConn1 -- upper_joint/LConn1
  shoulder_original/LConn1 -- shoulder_joint/RConn1
  "s_joint_ctrl "/LConn1 -- shoulder_joint/RConn2
  "s_joint_ctrl "/RConn1 -- shoulder_joint/LConn2
  "s_joint_ctrl "/LConn2 -- shoulder_joint/RConn3
  upper_joint/RConn2 -- "u_joint_ctrl "/LConn1
  upper_joint/LConn2 -- "u_joint_ctrl "/RConn1
  upper_joint/RConn3 -- "u_joint_ctrl "/LConn2
  knee_joint/RConn2 -- k_joint_ctrl/LConn1
  knee_joint/RConn3 -- k_joint_ctrl/LConn2
  k_joint_ctrl/RConn1 -- knee_joint/LConn2
  shoulder_torque/LConn1 -- shoulder_joint/RConn4
  upper_torque/LConn1 -- upper_joint/RConn4
  knee_torque/LConn1 -- knee_joint/RConn4

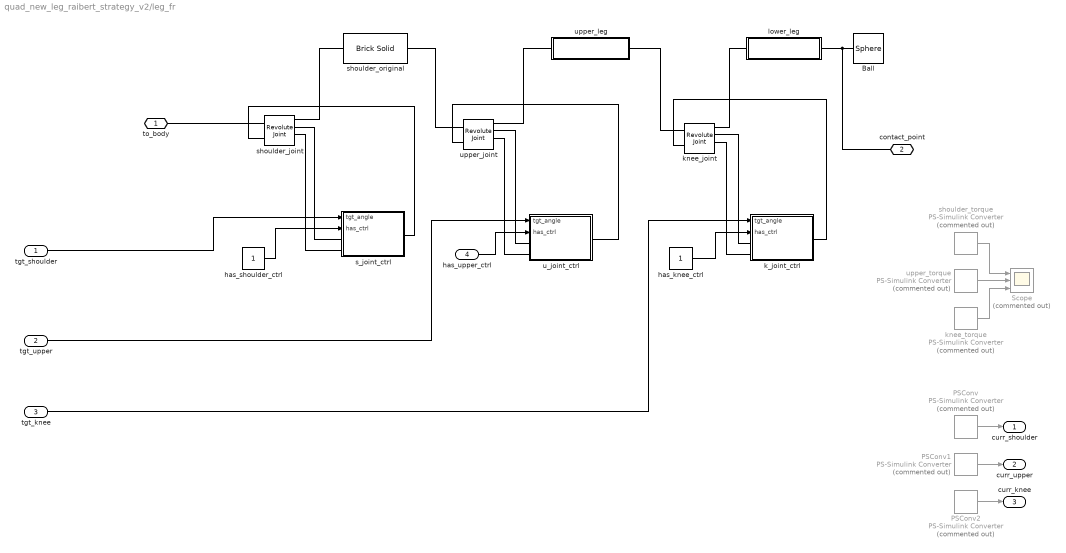
== system quad_new_leg_raibert_strategy_v2/leg_fr ==
  tgt_shoulder : Inport
  tgt_upper : Inport  Port=2
  tgt_knee : Inport  Port=3
  has_upper_ctrl : Inport  Port=4
  Ball : Parts_Lib/Sphere  Tag=CustomStyle  sph_radius=body.foot_radius  sph_density=1000  sph_color=red  sph_opacity=1  mark_type=Rings on center planes  arc_width=[40 50]  arc_angle=60  ring_width=5  ring_irad=0.95  mark_color=axes  mark_opacity=1  ring_opacity=0  arc_opacity=0
  PSConv : nesl_utility/PS-Simulink Converter  Commented=on  PhysicalDomain=network_engine_domain  SubClassName=ps_output  LeftPortType=input  RightPortType=output  PseudoPeriodic=off  Frequencies=[]  VectorFormat=1-D array  Unit=1  AffineConversion=off
  PSConv1 : nesl_utility/PS-Simulink Converter  Commented=on  PhysicalDomain=network_engine_domain  SubClassName=ps_output  LeftPortType=input  RightPortType=output  PseudoPeriodic=off  Frequencies=[]  VectorFormat=1-D array  Unit=1  AffineConversion=off
  PSConv2 : nesl_utility/PS-Simulink Converter  Commented=on  PhysicalDomain=network_engine_domain  SubClassName=ps_output  LeftPortType=input  RightPortType=output  PseudoPeriodic=off  Frequencies=[]  VectorFormat=1-D array  Unit=1  AffineConversion=off
  Scope : Scope  Commented=on  NumInputPorts=3
  "has_knee_ctrl " : Constant
  has_shoulder_ctrl : Constant
  k_joint_ctrl : Subsystem
  knee_joint : sm_lib/Joints/Revolute Joint  JointMode=Normal  SenseConstraintForce=off  SenseConstraintForceX=off  SenseConstraintForceY=off  SenseConstraintForceZ=off  SenseConstraintTorque=off  SenseConstraintTorqueX=off  SenseConstraintTorqueY=off  SenseConstraintTorqueZ=off  SenseTotalForce=off  SenseTotalForceX=off  SenseTotalForceY=off  SenseTotalForceZ=off  SenseTotalTorque=off  SenseTotalTorqueX=off  SenseTotalTorqueY=off  SenseTotalTorqueZ=off  CompositeWrenchDir=FollowerOnBase  CompositeWrenchFrame=BaseFrame  EquilibriumPosition=0  EquilibriumPositionUnits=deg  SpringStiffness=0  SpringStiffnessUnits=N*m/rad  DampingCoefficient=body.knee_damping  DampingCoefficientUnits=N*m/(deg/s)  TorqueActuationMode=InputTorque  MotionActuationMode=ComputedMotion  SensePosition=on  SenseVelocity=on  SenseAcceleration=off  SenseTorqueForce=on  SenseLowerLimitTorqueForce=off  SenseUpperLimitTorqueForce=off  LowerLimitSpecify=off  LowerLimitBound=-90  LowerLimitBoundUnits=deg  LowerLimitStiffness=1e4  LowerLimitStiffnessUnits=N*m/deg  LowerLimitDamping=10  LowerLimitDampingUnits=N*m/(deg/s)  LowerLimitTransitionRegionWidth=0.1  LowerLimitTransitionRegionWidthUnits=deg  UpperLimitSpecify=off  UpperLimitBound=90  UpperLimitBoundUnits=deg  UpperLimitStiffness=1e4  UpperLimitStiffnessUnits=N*m/deg  UpperLimitDamping=10  UpperLimitDampingUnits=N*m/(deg/s)  UpperLimitTransitionRegionWidth=0.1  UpperLimitTransitionRegionWidthUnits=deg  PositionTargetSpecify=off  PositionTargetPriority=High  PositionTargetValue=0  PositionTargetValueUnits=deg  VelocityTargetSpecify=off  VelocityTargetPriority=High  VelocityTargetValue=0  VelocityTargetValueUnits=deg/s
  knee_torque : nesl_utility/PS-Simulink Converter  Commented=on  PhysicalDomain=network_engine_domain  SubClassName=ps_output  LeftPortType=input  RightPortType=output  PseudoPeriodic=off  Frequencies=[]  VectorFormat=1-D array  Unit=1  AffineConversion=off
  lower_leg : Subsystem
  "s_joint_ctrl " : Subsystem
  shoulder_joint : sm_lib/Joints/Revolute Joint  JointMode=Normal  SenseConstraintForce=off  SenseConstraintForceX=off  SenseConstraintForceY=off  SenseConstraintForceZ=off  SenseConstraintTorque=off  SenseConstraintTorqueX=off  SenseConstraintTorqueY=off  SenseConstraintTorqueZ=off  SenseTotalForce=off  SenseTotalForceX=off  SenseTotalForceY=off  SenseTotalForceZ=off  SenseTotalTorque=off  SenseTotalTorqueX=off  SenseTotalTorqueY=off  SenseTotalTorqueZ=off  CompositeWrenchDir=FollowerOnBase  CompositeWrenchFrame=BaseFrame  EquilibriumPosition=0  EquilibriumPositionUnits=deg  SpringStiffness=0  SpringStiffnessUnits=N*m/deg  DampingCoefficient=0  DampingCoefficientUnits=N*m/(deg/s)  TorqueActuationMode=InputTorque  MotionActuationMode=ComputedMotion  SensePosition=on  SenseVelocity=on  SenseAcceleration=off  SenseTorqueForce=on  SenseLowerLimitTorqueForce=off  SenseUpperLimitTorqueForce=off  LowerLimitSpecify=off  LowerLimitBound=-90  LowerLimitBoundUnits=deg  LowerLimitStiffness=1e4  LowerLimitStiffnessUnits=N*m/deg  LowerLimitDamping=10  LowerLimitDampingUnits=N*m/(deg/s)  LowerLimitTransitionRegionWidth=0.1  LowerLimitTransitionRegionWidthUnits=deg  UpperLimitSpecify=off  UpperLimitBound=90  UpperLimitBoundUnits=deg  UpperLimitStiffness=1e4  UpperLimitStiffnessUnits=N*m/deg  UpperLimitDamping=10  UpperLimitDampingUnits=N*m/(deg/s)  UpperLimitTransitionRegionWidth=0.1  UpperLimitTransitionRegionWidthUnits=deg  PositionTargetSpecify=off  PositionTargetPriority=High  PositionTargetValue=0  PositionTargetValueUnits=deg  VelocityTargetSpecify=off  VelocityTargetPriority=High  VelocityTargetValue=0  VelocityTargetValueUnits=deg/s
  shoulder_original : sm_lib/Body Elements/Brick Solid  GraphicAmbientColor=[0.15 0.15 0.15 1.0]  BasedOnType=Density  BrickDimensions=[body.shoulder_size body.shoulder_size body.shoulder_size]  BrickDimensionUnits=m  CenterOfMass=[0 0 0]  CenterOfMassUnits=m  GraphicDiffuseColor=[0.2 0.4 0.6]  Density=660  DensityUnits=kg/(m^3)  DoExposeReferenceFrame=off  GraphicEmissiveColor=[0.0 0.0 0.0 1.0]  ExportEntireGeometry=off  SerializedFrames=<Frames><Frame><Id>Frame1</Id><Value><Name>to_body</Name><Origin><Source>CenterOfMassFrame</Source><FeatureName></FeatureName></Origin><PrimaryAxis><DefinedDirection>+Z</DefinedDirection><Source>ReferenceFrame</Source><SourceDirection>+X</SourceDirection><FeatureName></FeatureName></PrimaryAxis><SecondaryAxis><DefinedDirection>+X</DefinedDirection><Source>ReferenceFrame</Source><SourceDirection>-Z</SourceDirection><FeatureName></FeatureName></SecondaryAxis></Value></Frame><Frame><Id>Frame2</Id><Value><Name>to_leg</Name><Origin><Source>ReferenceFrame</Source><FeatureName></FeatureName></Origin><PrimaryAxis><DefinedDirection>+Z</DefinedDirection><Source>ReferenceFrame</Source><SourceDirection>+Y</SourceDirection><FeatureName></FeatureName></PrimaryAxis><SecondaryAxis><DefinedDirection>+X</DefinedDirection><Source>ReferenceFrame</Source><SourceDirection>+X</SourceDirection><FeatureName></FeatureName></SecondaryAxis></Value></Frame></Frames>  MarkerShape=Sphere  MarkerSize=10  GraphicType=FromGeometry  InertiaType=CalculateFromGeometry  Mass=1  MassUnits=kg  MomentsOfInertia=[1 1 1]  MomentsOfInertiaUnits=kg*m^2  GraphicOpacity=1.0  ProductsOfInertia=[0 0 0]  ProductsOfInertiaUnits=kg*m^2  GraphicShininess=75  GraphicSpecularColor=[0.5 0.5 0.5 1.0]  GraphicVisPropType=SimpleVisualProperties
  shoulder_torque : nesl_utility/PS-Simulink Converter  Commented=on  PhysicalDomain=network_engine_domain  SubClassName=ps_output  LeftPortType=input  RightPortType=output  PseudoPeriodic=off  Frequencies=[]  VectorFormat=1-D array  Unit=1  AffineConversion=off
  "u_joint_ctrl " : Subsystem
  upper_joint : sm_lib/Joints/Revolute Joint  JointMode=Normal  SenseConstraintForce=off  SenseConstraintForceX=off  SenseConstraintForceY=off  SenseConstraintForceZ=off  SenseConstraintTorque=off  SenseConstraintTorqueX=off  SenseConstraintTorqueY=off  SenseConstraintTorqueZ=off  SenseTotalForce=off  SenseTotalForceX=off  SenseTotalForceY=off  SenseTotalForceZ=off  SenseTotalTorque=off  SenseTotalTorqueX=off  SenseTotalTorqueY=off  SenseTotalTorqueZ=off  CompositeWrenchDir=FollowerOnBase  CompositeWrenchFrame=BaseFrame  EquilibriumPosition=0  EquilibriumPositionUnits=deg  SpringStiffness=0  SpringStiffnessUnits=N*m/deg  DampingCoefficient=0  DampingCoefficientUnits=N*m/(deg/s)  TorqueActuationMode=InputTorque  MotionActuationMode=ComputedMotion  SensePosition=on  SenseVelocity=on  SenseAcceleration=off  SenseTorqueForce=on  SenseLowerLimitTorqueForce=off  SenseUpperLimitTorqueForce=off  LowerLimitSpecify=off  LowerLimitBound=-90  LowerLimitBoundUnits=deg  LowerLimitStiffness=1e4  LowerLimitStiffnessUnits=N*m/deg  LowerLimitDamping=10  LowerLimitDampingUnits=N*m/(deg/s)  LowerLimitTransitionRegionWidth=0.1  LowerLimitTransitionRegionWidthUnits=deg  UpperLimitSpecify=off  UpperLimitBound=90  UpperLimitBoundUnits=deg  UpperLimitStiffness=1e4  UpperLimitStiffnessUnits=N*m/deg  UpperLimitDamping=10  UpperLimitDampingUnits=N*m/(deg/s)  UpperLimitTransitionRegionWidth=0.1  UpperLimitTransitionRegionWidthUnits=deg  PositionTargetSpecify=off  PositionTargetPriority=High  PositionTargetValue=0  PositionTargetValueUnits=deg  VelocityTargetSpecify=off  VelocityTargetPriority=High  VelocityTargetValue=0  VelocityTargetValueUnits=deg/s
  upper_leg : Subsystem
  upper_torque : nesl_utility/PS-Simulink Converter  Commented=on  PhysicalDomain=network_engine_domain  SubClassName=ps_output  LeftPortType=input  RightPortType=output  PseudoPeriodic=off  Frequencies=[]  VectorFormat=1-D array  Unit=1  AffineConversion=off
  to_body : PMIOPort  Side=Left
  contact_point : PMIOPort  Port=2  Side=Right
  curr_shoulder : Outport  VectorParamsAs1DForOutWhenUnconnected=off
  "curr_upper " : Outport  Port=2  VectorParamsAs1DForOutWhenUnconnected=off
  curr_knee : Outport  Port=3  VectorParamsAs1DForOutWhenUnconnected=off
  wires:
  "has_knee_ctrl "/1 -> k_joint_ctrl/2(has_ctrl)
  has_upper_ctrl/1 -> "u_joint_ctrl "/2(has_ctrl)
  has_shoulder_ctrl/1 -> "s_joint_ctrl "/2(has_ctrl)
  tgt_knee/1 -> k_joint_ctrl/1(tgt_angle)
  tgt_upper/1 -> "u_joint_ctrl "/1(tgt_angle)
  tgt_shoulder/1 -> "s_joint_ctrl "/1(tgt_angle)
  knee_torque/1 -> Scope/3
  upper_torque/1 -> Scope/2
  shoulder_torque/1 -> Scope/1
  PSConv2/1 -> curr_knee/1
  PSConv1/1 -> "curr_upper "/1
  PSConv/1 -> curr_shoulder/1
  connections:
  k_joint_ctrl/RConn1 -- knee_joint/LConn2
  knee_joint/RConn3 -- k_joint_ctrl/LConn2
  knee_joint/RConn2 -- k_joint_ctrl/LConn1
  upper_joint/RConn3 -- "u_joint_ctrl "/LConn2
  upper_joint/LConn2 -- "u_joint_ctrl "/RConn1
  upper_joint/RConn2 -- "u_joint_ctrl "/LConn1
  "s_joint_ctrl "/LConn2 -- shoulder_joint/RConn3
  "s_joint_ctrl "/RConn1 -- shoulder_joint/LConn2
  "s_joint_ctrl "/LConn1 -- shoulder_joint/RConn2
  shoulder_original/LConn1 -- shoulder_joint/RConn1
  shoulder_original/RConn1 -- upper_joint/LConn1
  to_body/RConn1 -- shoulder_joint/LConn1
  lower_leg/RConn1 -- knee_joint/RConn1
  upper_leg/LConn1 -- knee_joint/LConn1
  upper_leg/RConn1 -- upper_joint/RConn1
  Ball/LConn1 -- lower_leg/LConn1 -- contact_point/RConn1
